simulink model "Model_Kinematic"  (R2021b)
settings: Solver=VariableStepAuto  StartTime=0.0  StopTime=10  RelTol=1e-3
StopFcn:
  | clc
  | 
  | pos_n=pos.signals.values;
  | Joint_pxn=join_px.signals.values;
  | Joint_pyn=join_py.signals.values;
  | Joint_pzn=join_pz.signals.values;
  | 
  | xe=pos_n(:,1);
  | ye=pos_n(:,2);
  | ze=pos_n(:,3);
  | for i=1:size(pos_n,1)
  | figure(1)
  | clf
  | plot3(xe(1:i),ye(1:i),ze(1:i),'b--','LineWidth',2)
  | hold on
  | plot3(Joint_pxn(i,:),Joint_pyn(i,:),Joint_pzn(i,:),'r-o','LineWidth',2,'MarkerFaceColor','g','MarkerSize',7)
  | view(56,48)
  | 
  | grid on
  | pause(0.1)
  | end
  | 
  | xlabel('x(m)')
  | ylabel('y(m)')
  | zlabel('z(m)')
values from neighbouring files (symbols this model uses):
  pos = [loc;orientation]    [Direct_Kinematic.m]
settings Model: Creator=HJokar  LastModifiedBy=pc
settings SolverCC: AlgebraicLoopSolver=TrustRegion
settings DataIOCC: ReturnWorkspaceOutputs=off
settings DebuggingCC: SFMachineParentedDataDiag=warning  ArithmeticOperatorsInVariantConditions=warning
settings SFSimCC: CustomCodeUndefinedFunction=UseInterfaceOnly

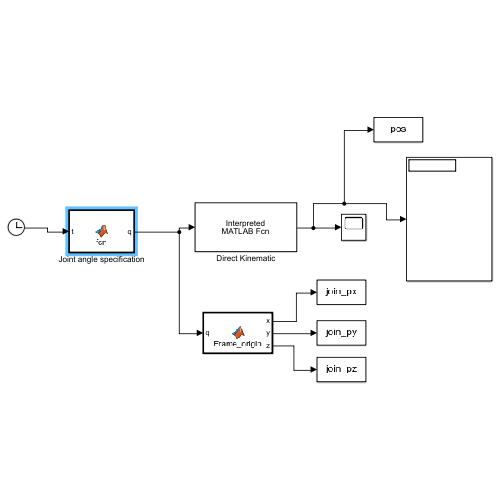
[thumbnail: Simulink's stored preview of the top-level diagram]
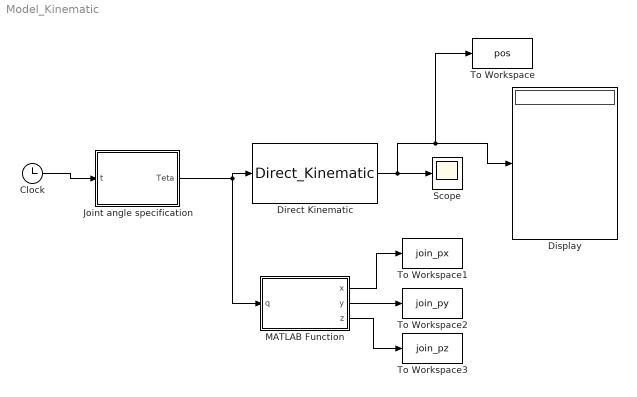
== system Model_Kinematic ==
  Clock : Clock
  Direct Kinematic : MATLABFcn  MATLABFcn=Direct_Kinematic  OutputSignalType=real
  Display : Display
  Joint angle specification : MATLAB Function  TreatAsAtomicUnit=on
  MATLAB Function : MATLAB Function  TreatAsAtomicUnit=on
  Scope : Scope
  To Workspace : ToWorkspace  VariableName=pos  SaveFormat=Structure With Time  SampleTime=-1
  To Workspace1 : ToWorkspace  VariableName=join_px  SaveFormat=Structure With Time  SampleTime=-1
  To Workspace2 : ToWorkspace  VariableName=join_py  SaveFormat=Structure With Time  SampleTime=-1
  To Workspace3 : ToWorkspace  VariableName=join_pz  SaveFormat=Structure With Time  SampleTime=-1
  wires:
  Direct Kinematic/1 -> To Workspace/1, Display/1, Scope/1
  Joint angle specification/1(Teta) -> Direct Kinematic/1, MATLAB Function/1(q)
  Clock/1 -> Joint angle specification/1(t)
  MATLAB Function/1(x) -> To Workspace1/1
  MATLAB Function/2(y) -> To Workspace2/1
  MATLAB Function/3(z) -> To Workspace3/1

== matlab function Model_Kinematic/MATLAB Function ==
  data: q input; x output; y output; z output
function [x,y,z]=Frame_origin(q)

nL=7;
d=[317*cos(asin(81/317)) 194.5 400 168.5 400 136.3 134.75]'*1e-3;
a=[0 81 0 0 0 0 0]'*1e-3; 
alpha=[0 -pi/2 -pi/2 -pi/2 pi/2 pi/2 -pi/2]';
teta=q;
teta(2)=teta(2)-pi/2;
Ti_im={zeros(4,4),zeros(4,4),zeros(4,4),zeros(4,4),zeros(4,4),zeros(4,4),zeros(4,4)};
Ti=Ti_im;
for i = 1:nL
    Ti_im{i} =[ cos(teta(i)) -sin(teta(i)) 0 a(i);
        sin(teta(i))*cos(alpha(i)) cos(teta(i))*cos(alpha(i)) -sin(alpha(i)) -sin(alpha(i))*d(i);
        sin(teta(i))*sin(alpha(i)) cos(teta(i))*sin(alpha(i)) cos(alpha(i)) cos(alpha(i))*d(i);
        0 0 0 1];
end
% 0_T_i
for i = 1:nL
    if i==1
        Ti{i}=Ti_im{i};
        
    else
        Ti{i}=Ti{i-1}*Ti_im{i};
    end
end
% Robot Configuration:

x=[0,Ti{1}(1,4) Ti{2}(1,4) Ti{3}(1,4) Ti{4}(1,4) Ti{5}(1,4) Ti{6}(1,4) Ti{7}(1,4)]';
y=[0,Ti{1}(2,4) Ti{2}(2,4) Ti{3}(2,4) Ti{4}(2,4) Ti{5}(2,4) Ti{6}(2,4) Ti{7}(2,4)]';
z=[0,Ti{1}(3,4) Ti{2}(3,4) Ti{3}(3,4) Ti{4}(3,4) Ti{5}(3,4) Ti{6}(3,4) Ti{7}(3,4)]';
end

== matlab function Model_Kinematic/Joint angle specification ==
  data: t input; Teta output
function Teta = fcn(t)
Teta=zeros(7,1);
Teta(1)=t;
Teta(2)=0;
Teta(3)=0;
Teta(4)=0;
Teta(5)=0;
Teta(6)=0;
Teta(7)=0;
